simulink model "Control"  (R2016a)
settings: Solver=VariableStepAuto  StartTime=0.0  StopTime=50  MaxStep=1e-3  RelTol=1e-3
libraries: nesl_utility x6, fl_lib x6, simulink x2
settings Model: Creator=AT Once  LastModifiedBy=maxha

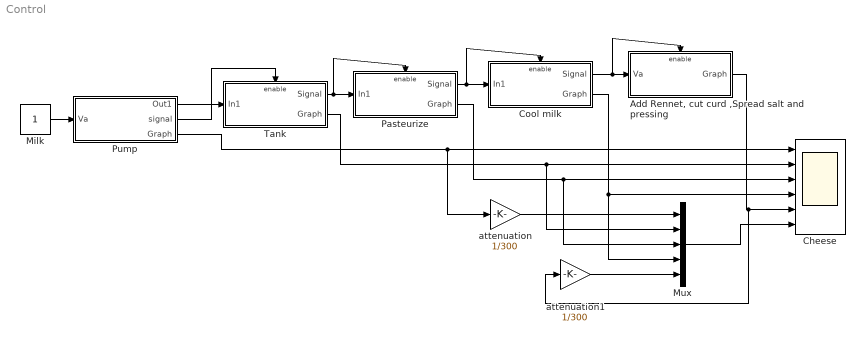
== system Control ==
  " Tank" : Subsystem
  "Add Rennet, cut curd ,Spread salt and pressing " : Subsystem
  Cheese : Scope  NumInputPorts=6
  Cool milk : Subsystem
  Milk : Constant
  Mux : Mux  Inputs=5
  Pasteurize : Subsystem
  "Pump " : Subsystem
  attenuation : Gain  Gain=1/300
  attenuation1 : Gain  Gain=1/300
  wires:
  Milk/1 -> "Pump "/1(Va)
  Mux/1 -> Cheese/6
  "Pump "/1(Out1) -> " Tank"/1(In1)
  " Tank"/1(Signal) -> Pasteurize/1(In1), Pasteurize/Enable
  Pasteurize/1(Signal) -> Cool milk/1(In1), Cool milk/Enable
  Cool milk/1(Signal) -> "Add Rennet, cut curd ,Spread salt and pressing "/Enable, "Add Rennet, cut curd ,Spread salt and pressing "/1(Va)
  "Pump "/2(signal) -> " Tank"/Enable
  "Add Rennet, cut curd ,Spread salt and pressing "/1(Graph) -> attenuation1/1, Cheese/5
  Cool milk/2(Graph) -> Mux/4, Cheese/4
  Pasteurize/2(Graph) -> Mux/3, Cheese/3
  " Tank"/2(Graph) -> Mux/2, Cheese/2
  "Pump "/3(Graph) -> attenuation/1, Cheese/1
  attenuation/1 -> Mux/1
  attenuation1/1 -> Mux/5

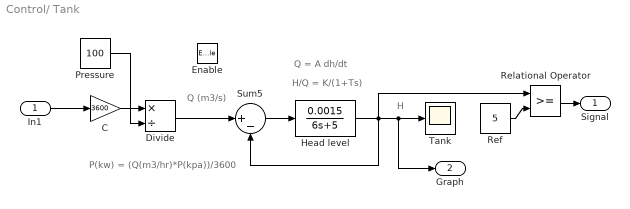
== system Control/ Tank ==
  note: Q = A dh/dt
  note: H/Q = K/(1+Ts)
  note: H
  note: Q (m3/s)
  note: P(kw) = (Q(m3/hr)*P(kpa))/3600
  In1 : Inport
  Enable : EnablePort
  C : Gain  Gain=3600
  Divide : Product  Inputs=*/
  "Head level " : TransferFcn  Numerator=[0.0015]  Denominator=[6 5]
  Pressure : Constant  Value=100
  Ref : Constant  Value=5
  Relational Operator : RelationalOperator  OutDataTypeStr=boolean
  Sum5 : Sum  Inputs=|+-
  Tank : Scope
  Signal : Outport
  Graph : Outport  Port=2
  wires:
  Divide/1 -> Sum5/1
  C/1 -> Divide/1
  Pressure/1 -> Divide/2
  Sum5/1 -> "Head level "/1
  In1/1 -> C/1
  "Head level "/1 -> Relational Operator/1, Graph/1, Tank/1, Sum5/2
  Ref/1 -> Relational Operator/2
  Relational Operator/1 -> Signal/1

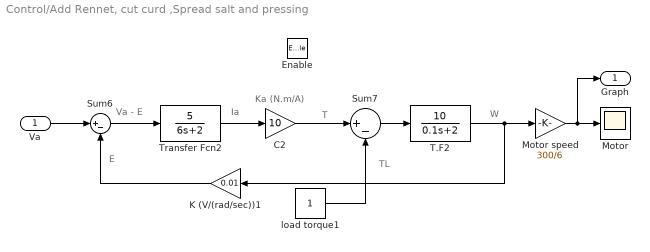
== system Control/Add Rennet, cut curd ,Spread salt and pressing  ==
  note: W
  note: TL
  note: T
  note: Ia
  note: Ka (N.m/A)
  note: E
  note: Va - E
  Va : Inport
  Enable : EnablePort
  C2 : Gain  Gain=10
  K (V/(rad/sec))1 : Gain  Gain=0.01
  Motor : Scope
  Motor speed : Gain  Gain=300/6
  Sum6 : Sum  Inputs=|+-
  Sum7 : Sum  Inputs=|+-
  T.F2 : TransferFcn  Numerator=[10]  Denominator=[0.1 2]
  Transfer Fcn2 : TransferFcn  Numerator=[5]  Denominator=[6 2]
  load torque1 : Constant
  Graph : Outport
  wires:
  Sum6/1 -> Transfer Fcn2/1
  Transfer Fcn2/1 -> C2/1
  Sum7/1 -> T.F2/1
  K (V/(rad/sec))1/1 -> Sum6/2
  load torque1/1 -> Sum7/2
  C2/1 -> Sum7/1
  Va/1 -> Sum6/1
  T.F2/1 -> K (V/(rad/sec))1/1, Motor speed/1
  Motor speed/1 -> Motor/1, Graph/1

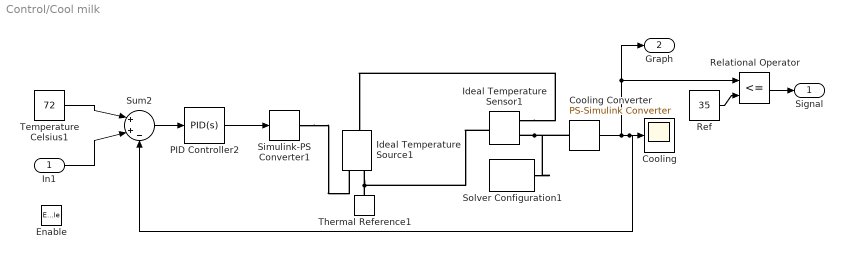
== system Control/Cool milk ==
  In1 : Inport
  Enable : EnablePort
  Cooling : Scope
  Cooling Converter : nesl_utility/PS-Simulink Converter  PhysicalDomain=network_engine_domain  SubClassName=ps_output  LeftPortType=input  RightPortType=output  PseudoPeriodic=off  Frequencies=[]  Unit=1  AffineConversion=off
  Ideal Temperature Sensor1 : fl_lib/Thermal/Thermal Sensors/Ideal Temperature Sensor
  Ideal Temperature Source1 : fl_lib/Thermal/Thermal Sources/Ideal Temperature Source
  PID Controller2 : simulink/Continuous/PID Controller  Controller=PID  TimeDomain=Continuous-time  SampleTime=-1  IntegratorMethod=Forward Euler  FilterMethod=Forward Euler  Form=Parallel  UseFilter=on  ControllerParametersSource=internal  P=-0.7  I=0  D=-5  N=100  InitialConditionSource=internal  InitialConditionForIntegrator=0  InitialConditionForFilter=0  ExternalReset=none  LimitOutput=off  UpperSaturationLimit=inf  LowerSaturationLimit=-inf  LinearizeAsGain=on  AntiWindupMode=none  Kb=1  TrackingMode=off  Kt=1  PParamMin=[]  PParamMax=[]  IParamMin=[]  IParamMax=[]  DParamMin=[]  DParamMax=[]  NParamMin=[]  NParamMax=[]  KbParamMin=[]  KbParamMax=[]  KtParamMin=[]  KtParamMax=[]  POutMin=[]  POutMax=[]  IOutMin=[]  IOutMax=[]  DOutMin=[]  DOutMax=[]  NOutMin=[]  NOutMax=[]  KbOutMin=[]  KbOutMax=[]  KtOutMin=[]  KtOutMax=[]  IntegratorOutMin=[]  IntegratorOutMax=[]  FilterOutMin=[]  FilterOutMax=[]  SumOutMin=[]  SumOutMax=[]  SumI1OutMin=[]  SumI1OutMax=[]  SumI2OutMin=[]  SumI2OutMax=[]  SumI3OutMin=[]  SumI3OutMax=[]  SumDOutMin=[]  SumDOutMax=[]  SaturationOutMin=[]  SaturationOutMax=[]  IntegratorContinuousStateAttributes=''  IntegratorStateMustResolveToSignalObject=off  IntegratorRTWStateStorageClass=Auto  FilterContinuousStateAttributes=''  FilterStateMustResolveToSignalObject=off  FilterRTWStateStorageClass=Auto  DifferentiatorICPrevScaledInput=0  DifferentiatorOutMin=[]  DifferentiatorOutMax=[]
  Ref : Constant  Value=35
  Relational Operator : RelationalOperator  Operator=<=  OutDataTypeStr=boolean
  Simulink-PS Converter1 : nesl_utility/Simulink-PS Converter  PhysicalDomain=network_engine_domain  SubClassName=ps_input  LeftPortType=input  RightPortType=output  PseudoPeriodic=off  Frequencies=[]  NoiseDistribution=none  NoiseParameters=[]  Unit=1  AffineConversion=off  InputFiltering=off  SimscapeFilterOrder=1  InputFilterTimeConstant=0.001  UdotUserProvided=1
  Solver Configuration1 : nesl_utility/Solver Configuration  PhysicalDomain=network_engine_domain  SubClassName=solver  LeftPortType=input  RightPortType=generic  Accelerate=off  Tones=[]  Harmonics=[]  SimulateNoise=off  Profile=off  UseLocalSampling=off  EnableSwitchedLinearOptims=on  FrequencyDomain=off  UseCCode=off  RelTol=0.001  AbsTol=1e-06  MinStep=1e-09  ToWorkspace=off  RevertToSquareIcSolve=off  NumHomotopyIterations=100  PhasorMode=off  PhasorModeNumHarmonics=1  OverrideAbsTol=off  DoDC=off  ResidualTolerance=1e-09  UseLocalSolver=off  LocalSolverChoice=NE_BACKWARD_EULER_ADVANCER  LocalSolverSampleTime=0.001  DoFixedCost=off  MaxNonlinIter=3  MaxModeIter=2  LinearAlgebra=Sparse  DelaysMemoryBudget=1024  AutomaticFiltering=on  FilteringTimeConstant=0.001
  Sum2 : Sum  Inputs=|++-
  Temperature Celsius1 : Constant  Value=72
  Thermal Reference1 : fl_lib/Thermal/Thermal Elements/Thermal Reference
  Signal : Outport
  Graph : Outport  Port=2
  wires:
  PID Controller2/1 -> Simulink-PS Converter1/1
  Sum2/1 -> PID Controller2/1
  Cooling Converter/1 -> Sum2/3, Cooling/1, Relational Operator/1, Graph/1
  Ref/1 -> Relational Operator/2
  Relational Operator/1 -> Signal/1
  Temperature Celsius1/1 -> Sum2/1
  In1/1 -> Sum2/2
  connections:
  Ideal Temperature Source1/RConn2 -- Ideal Temperature Sensor1/LConn1 -- Thermal Reference1/LConn1
  Ideal Temperature Sensor1/RConn2 -- Solver Configuration1/RConn1 -- Cooling Converter/LConn1
  Simulink-PS Converter1/RConn1 -- Ideal Temperature Source1/RConn1
  Ideal Temperature Sensor1/RConn1 -- Ideal Temperature Source1/LConn1

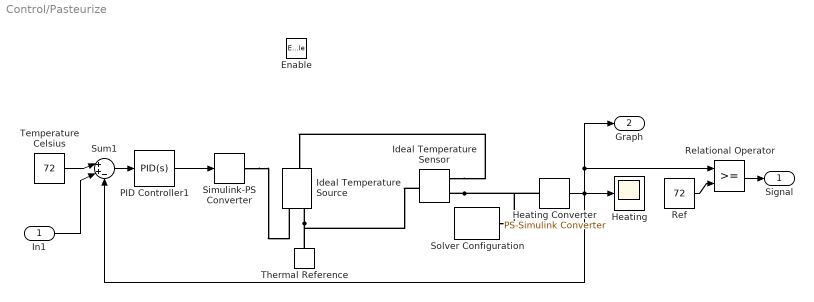
== system Control/Pasteurize ==
  In1 : Inport
  Enable : EnablePort
  Heating : Scope
  Heating Converter : nesl_utility/PS-Simulink Converter  PhysicalDomain=network_engine_domain  SubClassName=ps_output  LeftPortType=input  RightPortType=output  PseudoPeriodic=off  Frequencies=[]  Unit=1  AffineConversion=off
  Ideal Temperature Sensor : fl_lib/Thermal/Thermal Sensors/Ideal Temperature Sensor
  Ideal Temperature Source : fl_lib/Thermal/Thermal Sources/Ideal Temperature Source
  PID Controller1 : simulink/Continuous/PID Controller  Controller=PID  TimeDomain=Continuous-time  SampleTime=-1  IntegratorMethod=Forward Euler  FilterMethod=Forward Euler  Form=Parallel  UseFilter=on  ControllerParametersSource=internal  P=0  I=-0.316227766016838  D=0  N=100  InitialConditionSource=internal  InitialConditionForIntegrator=0  InitialConditionForFilter=0  ExternalReset=none  LimitOutput=off  UpperSaturationLimit=inf  LowerSaturationLimit=-inf  LinearizeAsGain=on  AntiWindupMode=none  Kb=1  TrackingMode=off  Kt=1  PParamMin=[]  PParamMax=[]  IParamMin=[]  IParamMax=[]  DParamMin=[]  DParamMax=[]  NParamMin=[]  NParamMax=[]  KbParamMin=[]  KbParamMax=[]  KtParamMin=[]  KtParamMax=[]  POutMin=[]  POutMax=[]  IOutMin=[]  IOutMax=[]  DOutMin=[]  DOutMax=[]  NOutMin=[]  NOutMax=[]  KbOutMin=[]  KbOutMax=[]  KtOutMin=[]  KtOutMax=[]  IntegratorOutMin=[]  IntegratorOutMax=[]  FilterOutMin=[]  FilterOutMax=[]  SumOutMin=[]  SumOutMax=[]  SumI1OutMin=[]  SumI1OutMax=[]  SumI2OutMin=[]  SumI2OutMax=[]  SumI3OutMin=[]  SumI3OutMax=[]  SumDOutMin=[]  SumDOutMax=[]  SaturationOutMin=[]  SaturationOutMax=[]  IntegratorContinuousStateAttributes=''  IntegratorStateMustResolveToSignalObject=off  IntegratorRTWStateStorageClass=Auto  FilterContinuousStateAttributes=''  FilterStateMustResolveToSignalObject=off  FilterRTWStateStorageClass=Auto  DifferentiatorICPrevScaledInput=0  DifferentiatorOutMin=[]  DifferentiatorOutMax=[]
  Ref : Constant  Value=72
  Relational Operator : RelationalOperator  OutDataTypeStr=boolean
  Simulink-PS Converter : nesl_utility/Simulink-PS Converter  PhysicalDomain=network_engine_domain  SubClassName=ps_input  LeftPortType=input  RightPortType=output  PseudoPeriodic=off  Frequencies=[]  NoiseDistribution=none  NoiseParameters=[]  Unit=1  AffineConversion=off  InputFiltering=off  SimscapeFilterOrder=1  InputFilterTimeConstant=0.001  UdotUserProvided=1
  Solver Configuration : nesl_utility/Solver Configuration  PhysicalDomain=network_engine_domain  SubClassName=solver  LeftPortType=input  RightPortType=generic  Accelerate=off  Tones=[]  Harmonics=[]  SimulateNoise=off  Profile=off  UseLocalSampling=off  EnableSwitchedLinearOptims=on  FrequencyDomain=off  UseCCode=off  RelTol=0.001  AbsTol=1e-06  MinStep=1e-09  ToWorkspace=off  RevertToSquareIcSolve=off  NumHomotopyIterations=100  PhasorMode=off  PhasorModeNumHarmonics=1  OverrideAbsTol=off  DoDC=off  ResidualTolerance=1e-09  UseLocalSolver=off  LocalSolverChoice=NE_BACKWARD_EULER_ADVANCER  LocalSolverSampleTime=0.001  DoFixedCost=off  MaxNonlinIter=3  MaxModeIter=2  LinearAlgebra=Sparse  DelaysMemoryBudget=1024  AutomaticFiltering=on  FilteringTimeConstant=0.001
  Sum1 : Sum  Inputs=|++-
  Temperature Celsius : Constant  Value=72
  Thermal Reference : fl_lib/Thermal/Thermal Elements/Thermal Reference
  Signal : Outport
  Graph : Outport  Port=2
  wires:
  Temperature Celsius/1 -> Sum1/1
  Sum1/1 -> PID Controller1/1
  PID Controller1/1 -> Simulink-PS Converter/1
  In1/1 -> Sum1/2
  Heating Converter/1 -> Heating/1, Sum1/3, Graph/1, Relational Operator/1
  Ref/1 -> Relational Operator/2
  Relational Operator/1 -> Signal/1
  connections:
  Ideal Temperature Source/RConn2 -- Thermal Reference/LConn1 -- Ideal Temperature Sensor/LConn1
  Ideal Temperature Sensor/RConn2 -- Heating Converter/LConn1 -- Solver Configuration/RConn1
  Simulink-PS Converter/RConn1 -- Ideal Temperature Source/RConn1
  Ideal Temperature Sensor/RConn1 -- Ideal Temperature Source/LConn1

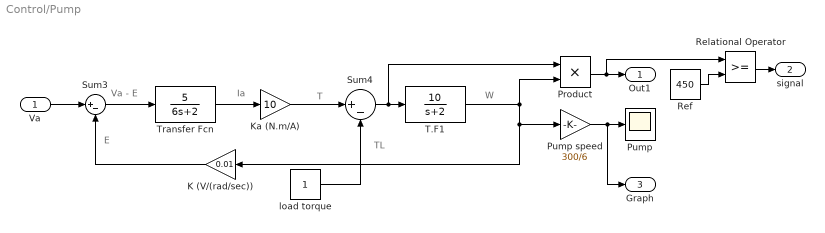
== system Control/Pump  ==
  note: W
  note: TL
  note: T
  note: Ia
  note: E
  note: Va - E
  Va : Inport
  K (V/(rad/sec)) : Gain  Gain=0.01
  Ka (N.m/A) : Gain  Gain=10
  Product : Product
  Pump : Scope
  Pump speed : Gain  Gain=300/6
  Ref : Constant  Value=450
  Relational Operator : RelationalOperator  OutDataTypeStr=boolean
  Sum3 : Sum  Inputs=|+-
  Sum4 : Sum  Inputs=|+-
  T.F1 : TransferFcn  Numerator=[10]  Denominator=[1 2]
  Transfer Fcn : TransferFcn  Numerator=[5]  Denominator=[6 2]
  load torque : Constant
  Out1 : Outport
  signal : Outport  Port=2
  Graph : Outport  Port=3
  wires:
  Sum3/1 -> Transfer Fcn/1
  Transfer Fcn/1 -> Ka (N.m/A)/1
  Sum4/1 -> Product/1, T.F1/1
  K (V/(rad/sec))/1 -> Sum3/2
  load torque/1 -> Sum4/2
  Ka (N.m/A)/1 -> Sum4/1
  Va/1 -> Sum3/1
  T.F1/1 -> Pump speed/1, K (V/(rad/sec))/1, Product/2
  Pump speed/1 -> Graph/1, Pump/1
  Product/1 -> Relational Operator/1, Out1/1
  Relational Operator/1 -> signal/1
  Ref/1 -> Relational Operator/2
